simulink model "VIPR557TrgtPos"  (R2018b)
settings: Solver=FixedStepDiscrete  StartTime=0.0  StopTime=10.0  RelTol=1e-3
settings Model: ModifiedHistory=2024.7.3 V3.0.0 557模式流程V1.9  Creator=sn2xws  LastModifiedBy=sn2xws
settings DataIOCC: SaveFormat=StructureWithTime
settings OptimizationCC: DefaultParameterBehavior=Inlined  EnhancedBackFolding=on  PassReuseOutputArgsAs=Individual arguments  ZeroExternalMemoryAtStartup=off  ZeroInternalMemoryAtStartup=off  OptimizeBlockOrder=speed  DifferentSizesBufferReuse=on  OptimizationCustomize=off
settings DebuggingCC: ParameterTunabilityLossMsg=error
settings SFSimCC: MATLABDynamicMemAlloc=off
settings RTWCC: SystemTargetFile=autosar.tlc  GenCodeOnly=on  TemplateMakefile=ert_default_tmf  Description=AUTOSAR  GenerateReport=on  IncludeHyperlinkInReport=on  LaunchReport=on  GenerateTraceInfo=on  GenerateTraceReport=on  GenerateTraceReportSl=on  GenerateTraceReportSf=on  GenerateTraceReportEml=on
settings CodeAppCC: ForceParamTrailComments=on  IgnoreCustomStorageClasses=off  OperatorAnnotations=on  SimulinkDataObjDesc=on  SFDataObjDesc=on  InsertBlockDesc=on
settings STFCustomTargetCC: TargetLangStandard=C99 (ISO)  MultiwordLength=256  ParMdlRefBuildCompliant=on  CompOptLevelCompliant=on  IncludeMdlTerminateFcn=off  CombineOutputUpdateFcns=on  SuppressErrorStatus=on  ERTCustomFileBanners=on  SupportNonFinite=off  SupportComplex=off  SupportContinuousTime=off  SupportNonInlinedSFcns=off  RemoveResetFunc=on  MATLABClassNameForMDSCustomization=Simulink.SoftwareTarget.ERTCustomization  AutosarCompliant=on  UseToolchainInfoCompliant=on  LookupTableObjectStructAxisOrder=2,1,3,4,...  LUTObjectStructOrderEvenSpacing=Size,Table,Breakpoints  SystemTargetFile=autosar.tlc
settings ERTTargetCC: TargetLangStandard=C99 (ISO)  ConcurrentExecutionCompliant=off  IncludeMdlTerminateFcn=off  SuppressErrorStatus=on  SupportNonFinite=off  SupportComplex=off  ModelStepFunctionPrototypeControlCompliant=off  CPPClassGenCompliant=off  AutosarCompliant=on  LookupTableObjectStructAxisOrder=2,1,3,4,...  LUTObjectStructOrderEvenSpacing=Size,Table,Breakpoints  InlinedParameterPlacement=NonHierarchical  ERTCustomFileTemplate=example_file_process.tlc  ERTFilePackagingFormat=Compact

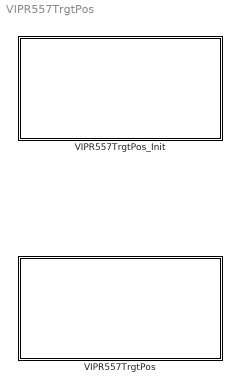
== system VIPR557TrgtPos ==
  VIPR557TrgtPos : Subsystem
  VIPR557TrgtPos_Init : Subsystem

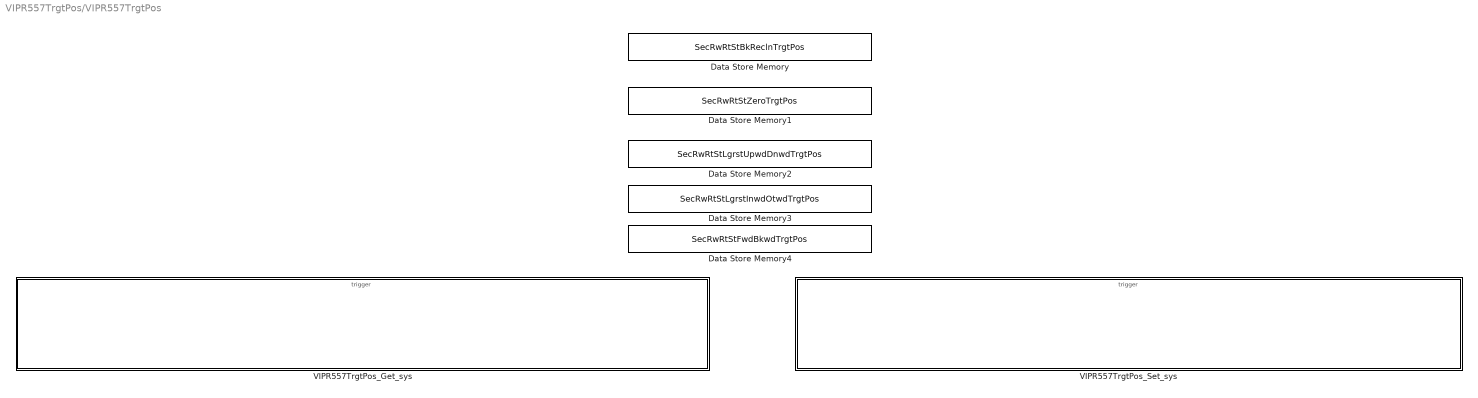
== system VIPR557TrgtPos/VIPR557TrgtPos ==
  Data Store Memory : DataStoreMemory  DataStoreName=SecRwRtStBkReclnTrgtPos  ReadBeforeWriteMsg=warning  WriteAfterWriteMsg=warning  WriteAfterReadMsg=warning  ShowAdditionalParam=off
  Data Store Memory1 : DataStoreMemory  DataStoreName=SecRwRtStZeroTrgtPos  ReadBeforeWriteMsg=warning  WriteAfterWriteMsg=warning  WriteAfterReadMsg=warning  ShowAdditionalParam=off
  Data Store Memory2 : DataStoreMemory  DataStoreName=SecRwRtStLgrstUpwdDnwdTrgtPos  ReadBeforeWriteMsg=warning  WriteAfterWriteMsg=warning  WriteAfterReadMsg=warning  ShowAdditionalParam=off
  Data Store Memory3 : DataStoreMemory  DataStoreName=SecRwRtStLgrstInwdOtwdTrgtPos  ReadBeforeWriteMsg=warning  WriteAfterWriteMsg=warning  WriteAfterReadMsg=warning  ShowAdditionalParam=off
  Data Store Memory4 : DataStoreMemory  DataStoreName=SecRwRtStFwdBkwdTrgtPos  ReadBeforeWriteMsg=warning  WriteAfterWriteMsg=warning  WriteAfterReadMsg=warning  ShowAdditionalParam=off
  VIPR557TrgtPos_Get_sys : Subsystem
  VIPR557TrgtPos_Set_sys : Subsystem

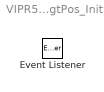
== system VIPR557TrgtPos/VIPR557TrgtPos_Init ==
  Event Listener : EventListener  EventName=reset

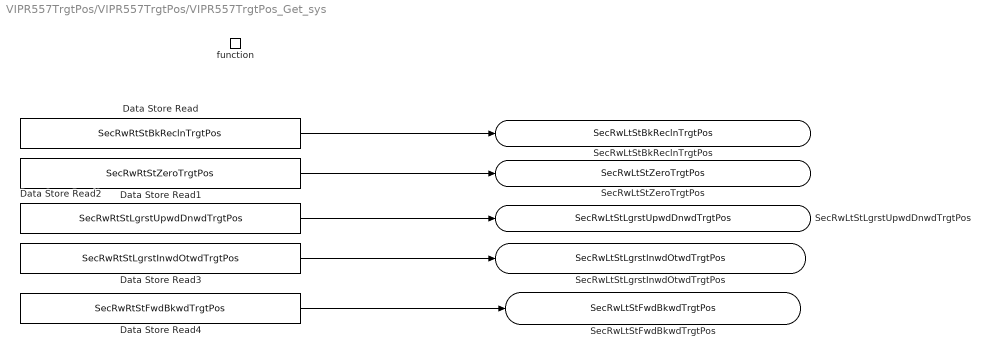
== system VIPR557TrgtPos/VIPR557TrgtPos/VIPR557TrgtPos_Get_sys ==
  function : TriggerPort  TriggerType=function-call  IsSimulinkFunction=on  FunctionName=VIPR557TrgtPos_Get  VariantControl=(inherit)
  Data Store Read : DataStoreRead  DataStoreName=SecRwRtStBkReclnTrgtPos
  Data Store Read1 : DataStoreRead  DataStoreName=SecRwRtStZeroTrgtPos
  Data Store Read2 : DataStoreRead  DataStoreName=SecRwRtStLgrstUpwdDnwdTrgtPos
  Data Store Read3 : DataStoreRead  DataStoreName=SecRwRtStLgrstInwdOtwdTrgtPos
  Data Store Read4 : DataStoreRead  DataStoreName=SecRwRtStFwdBkwdTrgtPos
  SecRwLtStBkReclnTrgtPos : ArgOut  OutDataTypeStr=uint16  ArgumentName=SecRwLtStBkReclnTrgtPos
  SecRwLtStZeroTrgtPos : ArgOut  Port=2  OutDataTypeStr=uint16  ArgumentName=SecRwLtStZeroTrgtPos
  SecRwLtStLgrstUpwdDnwdTrgtPos : ArgOut  Port=3  OutDataTypeStr=uint16  ArgumentName=SecRwLtStLgrstUpwdDnwdTrgtPos
  SecRwLtStLgrstInwdOtwdTrgtPos : ArgOut  Port=4  OutDataTypeStr=uint16  ArgumentName=SecRwLtStLgrstInwdOtwdTrgtPos
  SecRwLtStFwdBkwdTrgtPos : ArgOut  Port=5  OutDataTypeStr=uint16  ArgumentName=SecRwLtStFwdBkwdTrgtPos
  wires:
  Data Store Read1/1 -> SecRwLtStZeroTrgtPos/1
  Data Store Read2/1 -> SecRwLtStLgrstUpwdDnwdTrgtPos/1
  Data Store Read3/1 -> SecRwLtStLgrstInwdOtwdTrgtPos/1
  Data Store Read/1 -> SecRwLtStBkReclnTrgtPos/1
  Data Store Read4/1 -> SecRwLtStFwdBkwdTrgtPos/1

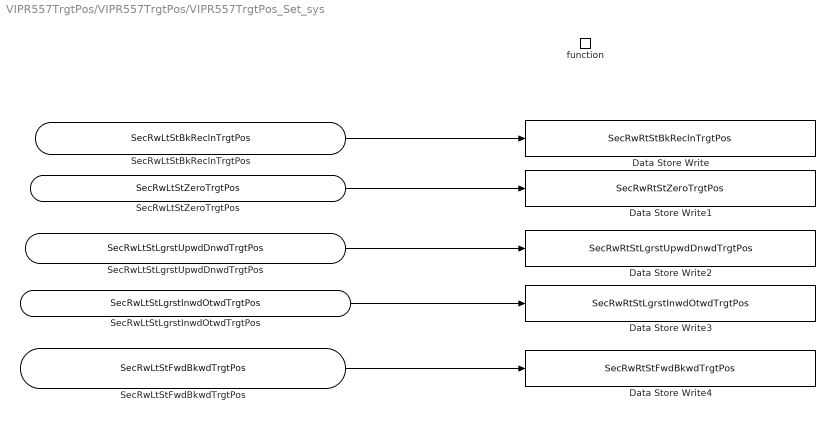
== system VIPR557TrgtPos/VIPR557TrgtPos/VIPR557TrgtPos_Set_sys ==
  function : TriggerPort  TriggerType=function-call  IsSimulinkFunction=on  FunctionName=VIPR557TrgtPos_Set  VariantControl=(inherit)
  Data Store Write : DataStoreWrite  DataStoreName=SecRwRtStBkReclnTrgtPos
  Data Store Write1 : DataStoreWrite  DataStoreName=SecRwRtStZeroTrgtPos
  Data Store Write2 : DataStoreWrite  DataStoreName=SecRwRtStLgrstUpwdDnwdTrgtPos
  Data Store Write3 : DataStoreWrite  DataStoreName=SecRwRtStLgrstInwdOtwdTrgtPos
  Data Store Write4 : DataStoreWrite  DataStoreName=SecRwRtStFwdBkwdTrgtPos
  SecRwLtStBkReclnTrgtPos : ArgIn  OutDataTypeStr=uint16  ArgumentName=SecRwLtStBkReclnTrgtPos
  SecRwLtStZeroTrgtPos : ArgIn  Port=2  OutDataTypeStr=uint16  ArgumentName=SecRwLtStZeroTrgtPos
  SecRwLtStLgrstUpwdDnwdTrgtPos : ArgIn  Port=3  OutDataTypeStr=uint16  ArgumentName=SecRwLtStLgrstUpwdDnwdTrgtPos
  SecRwLtStLgrstInwdOtwdTrgtPos : ArgIn  Port=4  OutDataTypeStr=uint16  ArgumentName=SecRwLtStLgrstInwdOtwdTrgtPos
  SecRwLtStFwdBkwdTrgtPos : ArgIn  Port=5  OutDataTypeStr=uint16  ArgumentName=SecRwLtStFwdBkwdTrgtPos
  wires:
  SecRwLtStLgrstUpwdDnwdTrgtPos/1 -> Data Store Write2/1
  SecRwLtStZeroTrgtPos/1 -> Data Store Write1/1
  SecRwLtStBkReclnTrgtPos/1 -> Data Store Write/1
  SecRwLtStLgrstInwdOtwdTrgtPos/1 -> Data Store Write3/1
  SecRwLtStFwdBkwdTrgtPos/1 -> Data Store Write4/1
